simulink model "example3"  (R2017a)
settings: Solver=FixedStepAuto  StartTime=0.0  StopTime=10.0  RelTol=1e-3
settings Model: Creator=rober  LastModifiedBy=rober
settings SolverCC: AutoInsertRateTranBlk=on

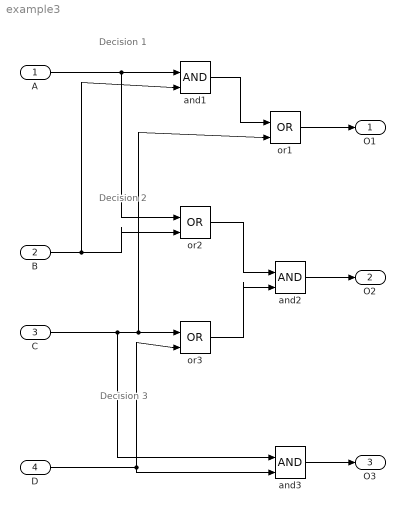
== system example3 ==
  note: Decision 3
  note: Decision 2
  note: Decision 1
  A : Inport  OutDataTypeStr=boolean
  B : Inport  Port=2  OutDataTypeStr=boolean
  C : Inport  Port=3  OutDataTypeStr=boolean
  D : Inport  Port=4  OutDataTypeStr=boolean
  and1 : Logic  IconShape=distinctive  AllPortsSameDT=off  OutDataTypeStr=boolean
  and2 : Logic  IconShape=distinctive  AllPortsSameDT=off  OutDataTypeStr=boolean
  and3 : Logic  IconShape=distinctive  AllPortsSameDT=off  OutDataTypeStr=boolean
  or1 : Logic  Operator=OR  IconShape=distinctive  AllPortsSameDT=off  OutDataTypeStr=boolean
  or2 : Logic  Operator=OR  IconShape=distinctive  AllPortsSameDT=off  OutDataTypeStr=boolean
  "or3 " : Logic  Operator=OR  IconShape=distinctive  AllPortsSameDT=off  OutDataTypeStr=boolean
  O1 : Outport
  O2 : Outport  Port=2
  O3 : Outport  Port=3
  wires:
  A/1 -> or2/1, and1/1
  B/1 -> and1/2, or2/2
  or2/1 -> and2/1
  and2/1 -> O2/1
  C/1 -> and3/1, or1/2, "or3 "/1
  D/1 -> and3/2, "or3 "/2
  "or3 "/1 -> and2/2
  or1/1 -> O1/1
  and1/1 -> or1/1
  and3/1 -> O3/1
